simulink model "Room5310Simulation_Aircondition"  (R2025b)
settings: Solver=VariableStepAuto  StartTime=0.0  StopTime=3600*3  RelTol=1e-3
model workspace (MAT data in the model file):
  Comp_eff = 0.85
  Dia_LiquidPipe = 3.17e-05
  Dia_SuctionPipe = 0.000196
  Q_Evap_Require = 22.86
libraries: fl_lib x57, nesl_utility x21, SimscapeFluids_lib x8
(part 2 of 2)

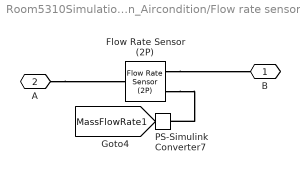
== system Room5310Simulation_Aircondition/Flow rate sensor 1 ==
  Flow Rate Sensor (2P) : fl_lib/Two-Phase Fluid/Sensors/Flow Rate Sensor (2P)  mass_flow_measure=true  volumetric_flow_measure=false  energy_flow_measure=false
      settings: InternalSimscapePortConfiguration="{\"Bottom\":[],\"Left\":[{\"id\":\"A\",\"label\":\"A\",\"type\":\"foundation.two_phase_fluid.two_phase_fluid\"}],\"Right\":[{\"id\":\"B\",\"label\":\"B\",\"type\":\"foundation.two_phase_fluid.two_phase_fluid\"},{\"id\":\"M\",\"label\":\"M\",\"type\":\"output\"}],\"Top\":[]}"
  PS-Simulink Converter7 : nesl_utility/PS-Simulink Converter  PhysicalDomain=network_engine_domain  SubClassName=ps_output  LeftPortType=input  RightPortType=output  PseudoPeriodic=off  Frequencies=[]  VectorFormat=inherit  Unit=inherit  AffineConversion=off
  B : PMIOPort  Side=Right
  A : PMIOPort  Port=2  Side=Left
  tag scope: MassFlowRate1=global
  wires:
  PS-Simulink Converter7/1 -> [MassFlowRate1]
  connections:
  Flow Rate Sensor (2P)/RConn2 -- PS-Simulink Converter7/LConn1
  Flow Rate Sensor (2P)/RConn1 -- B/RConn1
  A/RConn1 -- Flow Rate Sensor (2P)/LConn1

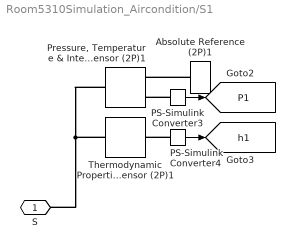
== system Room5310Simulation_Aircondition/S1 ==
  Absolute Reference (2P)1 : fl_lib/Two-Phase Fluid/Elements/Absolute Reference (2P)
  PS-Simulink Converter3 : nesl_utility/PS-Simulink Converter  PhysicalDomain=network_engine_domain  SubClassName=ps_output  LeftPortType=input  RightPortType=output  PseudoPeriodic=off  Frequencies=[]  VectorFormat=inherit  Unit=inherit  AffineConversion=off
  PS-Simulink Converter4 : nesl_utility/PS-Simulink Converter  PhysicalDomain=network_engine_domain  SubClassName=ps_output  LeftPortType=input  RightPortType=output  PseudoPeriodic=off  Frequencies=[]  VectorFormat=inherit  Unit=inherit  AffineConversion=off
  "Pressure, Temperature & Internal Energy Sensor (2P)1" : fl_lib/Two-Phase Fluid/Sensors/Pressure, Temperature & Internal Energy Sensor (2P)  reference=foundation.enum.MeasurementReference.difference  pressure=true  pressure_spec=foundation.enum.PressureMeasementSpec.Absolute  temperature=false  internal_energy=false
      settings: InternalSimscapePortConfiguration="{\"Bottom\":[],\"Left\":[{\"id\":\"A\",\"label\":\"A\",\"type\":\"foundation.two_phase_fluid.two_phase_fluid\"}],\"Right\":[{\"id\":\"B\",\"label\":\"B\",\"type\":\"foundation.two_phase_fluid.two_phase_fluid\"},{\"id\":\"P\",\"label\":\"P\",\"type\":\"output\"}],\"Top\":[]}"
  Thermodynamic Properties Sensor (2P)1 : fl_lib/Two-Phase Fluid/Sensors/Thermodynamic Properties Sensor (2P)  temperature=false  enthalpy=true  density=false  specific_volume=false  entropy=false
      settings: InternalSimscapePortConfiguration="{\"Bottom\":[],\"Left\":[{\"id\":\"A\",\"label\":\"A\",\"type\":\"foundation.two_phase_fluid.two_phase_fluid\"}],\"Right\":[{\"id\":\"H\",\"label\":\"h\",\"type\":\"output\"}],\"Top\":[]}"
  S : PMIOPort  Side=Right
  tag scope: P1=global, h1=global
  wires:
  PS-Simulink Converter4/1 -> [h1]
  PS-Simulink Converter3/1 -> [P1]
  connections:
  Thermodynamic Properties Sensor (2P)1/LConn1 -- S/RConn1 -- "Pressure, Temperature & Internal Energy Sensor (2P)1"/LConn1
  Absolute Reference (2P)1/LConn1 -- "Pressure, Temperature & Internal Energy Sensor (2P)1"/RConn1
  PS-Simulink Converter4/LConn1 -- Thermodynamic Properties Sensor (2P)1/RConn1
  PS-Simulink Converter3/LConn1 -- "Pressure, Temperature & Internal Energy Sensor (2P)1"/RConn2

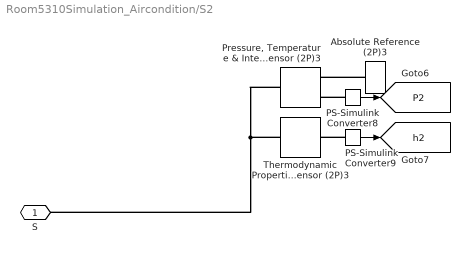
== system Room5310Simulation_Aircondition/S2 ==
  Absolute Reference (2P)3 : fl_lib/Two-Phase Fluid/Elements/Absolute Reference (2P)
  PS-Simulink Converter8 : nesl_utility/PS-Simulink Converter  PhysicalDomain=network_engine_domain  SubClassName=ps_output  LeftPortType=input  RightPortType=output  PseudoPeriodic=off  Frequencies=[]  VectorFormat=inherit  Unit=inherit  AffineConversion=off
  PS-Simulink Converter9 : nesl_utility/PS-Simulink Converter  PhysicalDomain=network_engine_domain  SubClassName=ps_output  LeftPortType=input  RightPortType=output  PseudoPeriodic=off  Frequencies=[]  VectorFormat=inherit  Unit=inherit  AffineConversion=off
  "Pressure, Temperature & Internal Energy Sensor (2P)3" : fl_lib/Two-Phase Fluid/Sensors/Pressure, Temperature & Internal Energy Sensor (2P)  reference=foundation.enum.MeasurementReference.difference  pressure=true  pressure_spec=foundation.enum.PressureMeasementSpec.Absolute  temperature=false  internal_energy=false
      settings: InternalSimscapePortConfiguration="{\"Bottom\":[],\"Left\":[{\"id\":\"A\",\"label\":\"A\",\"type\":\"foundation.two_phase_fluid.two_phase_fluid\"}],\"Right\":[{\"id\":\"B\",\"label\":\"B\",\"type\":\"foundation.two_phase_fluid.two_phase_fluid\"},{\"id\":\"P\",\"label\":\"P\",\"type\":\"output\"}],\"Top\":[]}"
  Thermodynamic Properties Sensor (2P)3 : fl_lib/Two-Phase Fluid/Sensors/Thermodynamic Properties Sensor (2P)  temperature=false  enthalpy=true  density=false  specific_volume=false  entropy=false
      settings: InternalSimscapePortConfiguration="{\"Bottom\":[],\"Left\":[{\"id\":\"A\",\"label\":\"A\",\"type\":\"foundation.two_phase_fluid.two_phase_fluid\"}],\"Right\":[{\"id\":\"H\",\"label\":\"h\",\"type\":\"output\"}],\"Top\":[]}"
  S : PMIOPort  Side=Left
  tag scope: P2=global, h2=global
  wires:
  PS-Simulink Converter8/1 -> [P2]
  PS-Simulink Converter9/1 -> [h2]
  connections:
  PS-Simulink Converter8/LConn1 -- "Pressure, Temperature & Internal Energy Sensor (2P)3"/RConn2
  PS-Simulink Converter9/LConn1 -- Thermodynamic Properties Sensor (2P)3/RConn1
  Absolute Reference (2P)3/LConn1 -- "Pressure, Temperature & Internal Energy Sensor (2P)3"/RConn1
  "Pressure, Temperature & Internal Energy Sensor (2P)3"/LConn1 -- S/RConn1 -- Thermodynamic Properties Sensor (2P)3/LConn1

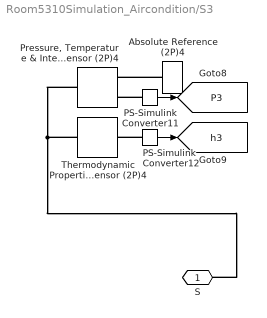
== system Room5310Simulation_Aircondition/S3 ==
  Absolute Reference (2P)4 : fl_lib/Two-Phase Fluid/Elements/Absolute Reference (2P)
  PS-Simulink Converter11 : nesl_utility/PS-Simulink Converter  PhysicalDomain=network_engine_domain  SubClassName=ps_output  LeftPortType=input  RightPortType=output  PseudoPeriodic=off  Frequencies=[]  VectorFormat=inherit  Unit=inherit  AffineConversion=off
  PS-Simulink Converter12 : nesl_utility/PS-Simulink Converter  PhysicalDomain=network_engine_domain  SubClassName=ps_output  LeftPortType=input  RightPortType=output  PseudoPeriodic=off  Frequencies=[]  VectorFormat=inherit  Unit=inherit  AffineConversion=off
  "Pressure, Temperature & Internal Energy Sensor (2P)4" : fl_lib/Two-Phase Fluid/Sensors/Pressure, Temperature & Internal Energy Sensor (2P)  reference=foundation.enum.MeasurementReference.difference  pressure=true  pressure_spec=foundation.enum.PressureMeasementSpec.Absolute  temperature=false  internal_energy=false
      settings: InternalSimscapePortConfiguration="{\"Bottom\":[],\"Left\":[{\"id\":\"A\",\"label\":\"A\",\"type\":\"foundation.two_phase_fluid.two_phase_fluid\"}],\"Right\":[{\"id\":\"B\",\"label\":\"B\",\"type\":\"foundation.two_phase_fluid.two_phase_fluid\"},{\"id\":\"P\",\"label\":\"P\",\"type\":\"output\"}],\"Top\":[]}"
  Thermodynamic Properties Sensor (2P)4 : fl_lib/Two-Phase Fluid/Sensors/Thermodynamic Properties Sensor (2P)  temperature=false  enthalpy=true  density=false  specific_volume=false  entropy=false
      settings: InternalSimscapePortConfiguration="{\"Bottom\":[],\"Left\":[{\"id\":\"A\",\"label\":\"A\",\"type\":\"foundation.two_phase_fluid.two_phase_fluid\"}],\"Right\":[{\"id\":\"H\",\"label\":\"h\",\"type\":\"output\"}],\"Top\":[]}"
  S : PMIOPort  Side=Right
  tag scope: P3=global, h3=global
  wires:
  PS-Simulink Converter11/1 -> [P3]
  PS-Simulink Converter12/1 -> [h3]
  connections:
  PS-Simulink Converter11/LConn1 -- "Pressure, Temperature & Internal Energy Sensor (2P)4"/RConn2
  Thermodynamic Properties Sensor (2P)4/LConn1 -- S/RConn1 -- "Pressure, Temperature & Internal Energy Sensor (2P)4"/LConn1
  PS-Simulink Converter12/LConn1 -- Thermodynamic Properties Sensor (2P)4/RConn1
  Absolute Reference (2P)4/LConn1 -- "Pressure, Temperature & Internal Energy Sensor (2P)4"/RConn1

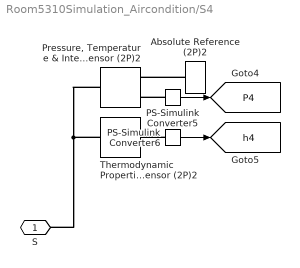
== system Room5310Simulation_Aircondition/S4 ==
  Absolute Reference (2P)2 : fl_lib/Two-Phase Fluid/Elements/Absolute Reference (2P)
  PS-Simulink Converter5 : nesl_utility/PS-Simulink Converter  PhysicalDomain=network_engine_domain  SubClassName=ps_output  LeftPortType=input  RightPortType=output  PseudoPeriodic=off  Frequencies=[]  VectorFormat=inherit  Unit=inherit  AffineConversion=off
  PS-Simulink Converter6 : nesl_utility/PS-Simulink Converter  PhysicalDomain=network_engine_domain  SubClassName=ps_output  LeftPortType=input  RightPortType=output  PseudoPeriodic=off  Frequencies=[]  VectorFormat=inherit  Unit=inherit  AffineConversion=off
  "Pressure, Temperature & Internal Energy Sensor (2P)2" : fl_lib/Two-Phase Fluid/Sensors/Pressure, Temperature & Internal Energy Sensor (2P)  reference=foundation.enum.MeasurementReference.difference  pressure=true  pressure_spec=foundation.enum.PressureMeasementSpec.Absolute  temperature=false  internal_energy=false
      settings: InternalSimscapePortConfiguration="{\"Bottom\":[],\"Left\":[{\"id\":\"A\",\"label\":\"A\",\"type\":\"foundation.two_phase_fluid.two_phase_fluid\"}],\"Right\":[{\"id\":\"B\",\"label\":\"B\",\"type\":\"foundation.two_phase_fluid.two_phase_fluid\"},{\"id\":\"P\",\"label\":\"P\",\"type\":\"output\"}],\"Top\":[]}"
  Thermodynamic Properties Sensor (2P)2 : fl_lib/Two-Phase Fluid/Sensors/Thermodynamic Properties Sensor (2P)  temperature=false  enthalpy=true  density=false  specific_volume=false  entropy=false
      settings: InternalSimscapePortConfiguration="{\"Bottom\":[],\"Left\":[{\"id\":\"A\",\"label\":\"A\",\"type\":\"foundation.two_phase_fluid.two_phase_fluid\"}],\"Right\":[{\"id\":\"H\",\"label\":\"h\",\"type\":\"output\"}],\"Top\":[]}"
  S : PMIOPort  Side=Right
  tag scope: P4=global, h4=global
  wires:
  PS-Simulink Converter6/1 -> [h4]
  PS-Simulink Converter5/1 -> [P4]
  connections:
  Absolute Reference (2P)2/LConn1 -- "Pressure, Temperature & Internal Energy Sensor (2P)2"/RConn1
  PS-Simulink Converter5/LConn1 -- "Pressure, Temperature & Internal Energy Sensor (2P)2"/RConn2
  PS-Simulink Converter6/LConn1 -- Thermodynamic Properties Sensor (2P)2/RConn1
  Thermodynamic Properties Sensor (2P)2/LConn1 -- S/RConn1 -- "Pressure, Temperature & Internal Energy Sensor (2P)2"/LConn1

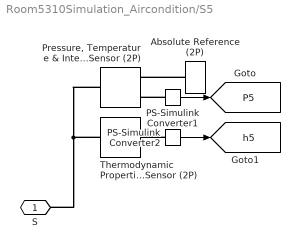
== system Room5310Simulation_Aircondition/S5 ==
  Absolute Reference (2P) : fl_lib/Two-Phase Fluid/Elements/Absolute Reference (2P)
  PS-Simulink Converter1 : nesl_utility/PS-Simulink Converter  PhysicalDomain=network_engine_domain  SubClassName=ps_output  LeftPortType=input  RightPortType=output  PseudoPeriodic=off  Frequencies=[]  VectorFormat=inherit  Unit=inherit  AffineConversion=off
  PS-Simulink Converter2 : nesl_utility/PS-Simulink Converter  PhysicalDomain=network_engine_domain  SubClassName=ps_output  LeftPortType=input  RightPortType=output  PseudoPeriodic=off  Frequencies=[]  VectorFormat=inherit  Unit=inherit  AffineConversion=off
  "Pressure, Temperature & Internal Energy Sensor (2P)" : fl_lib/Two-Phase Fluid/Sensors/Pressure, Temperature & Internal Energy Sensor (2P)  reference=foundation.enum.MeasurementReference.difference  pressure=true  pressure_spec=foundation.enum.PressureMeasementSpec.Absolute  temperature=false  internal_energy=false
      settings: InternalSimscapePortConfiguration="{\"Bottom\":[],\"Left\":[{\"id\":\"A\",\"label\":\"A\",\"type\":\"foundation.two_phase_fluid.two_phase_fluid\"}],\"Right\":[{\"id\":\"B\",\"label\":\"B\",\"type\":\"foundation.two_phase_fluid.two_phase_fluid\"},{\"id\":\"P\",\"label\":\"P\",\"type\":\"output\"}],\"Top\":[]}"
  Thermodynamic Properties Sensor (2P) : fl_lib/Two-Phase Fluid/Sensors/Thermodynamic Properties Sensor (2P)  temperature=false  enthalpy=true  density=false  specific_volume=false  entropy=false
      settings: InternalSimscapePortConfiguration="{\"Bottom\":[],\"Left\":[{\"id\":\"A\",\"label\":\"A\",\"type\":\"foundation.two_phase_fluid.two_phase_fluid\"}],\"Right\":[{\"id\":\"H\",\"label\":\"h\",\"type\":\"output\"}],\"Top\":[]}"
  S : PMIOPort  Side=Left
  tag scope: P5=global, h5=global
  wires:
  PS-Simulink Converter1/1 -> [P5]
  PS-Simulink Converter2/1 -> [h5]
  connections:
  PS-Simulink Converter1/LConn1 -- "Pressure, Temperature & Internal Energy Sensor (2P)"/RConn2
  PS-Simulink Converter2/LConn1 -- Thermodynamic Properties Sensor (2P)/RConn1
  "Pressure, Temperature & Internal Energy Sensor (2P)"/LConn1 -- S/RConn1 -- Thermodynamic Properties Sensor (2P)/LConn1
  Absolute Reference (2P)/LConn1 -- "Pressure, Temperature & Internal Energy Sensor (2P)"/RConn1

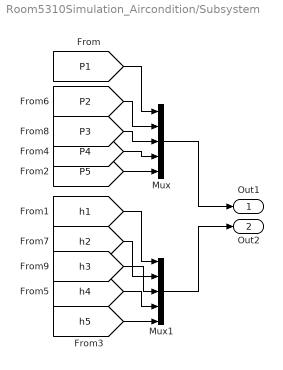
== system Room5310Simulation_Aircondition/Subsystem ==
  Mux : Mux  Inputs=5
  Mux1 : Mux  Inputs=5
  Out1 : Outport
  Out2 : Outport  Port=2
  wires:
  [h4] -> Mux1/4
  [h5] -> Mux1/5
  [P2] -> Mux/2
  [h1] -> Mux1/1
  [P1] -> Mux/1
  [h2] -> Mux1/2
  Mux1/1 -> Out2/1
  [h3] -> Mux1/3
  [P4] -> Mux/4
  [P3] -> Mux/3
  [P5] -> Mux/5
  Mux/1 -> Out1/1
